simulink model "closeloop2PIBC"  (R2021a)
settings: Solver=VariableStepAuto  StartTime=0.0  StopTime=0.5  FixedStep=1e-7  MaxStep=1e-6  RelTol=1e-3
PreLoadFcn:
  | L=32e-6;
  | k=-1/3;
  | M=  L*k
  | %N=4 %nbre de spires
  | rL=3.34e-3;
  | V_dc=14.4;
  | C=100e-6;
  | r_load=5;
undefined symbols (not defined in the file or in its folder): plecs
settings Model: Creator=QUDUS  LastModifiedBy=qaromose
settings DebuggingCC: UnconnectedInputMsg=none  UnconnectedOutputMsg=none  UnconnectedLineMsg=none
settings ModelReferenceCC: EnableRefExpFcnMdlSchedulingChecks=off
settings RTWCC: Description=Generic Real-Time Target  GPUComputeCapability=5.0  DLArmComputeVersion=20.02.1

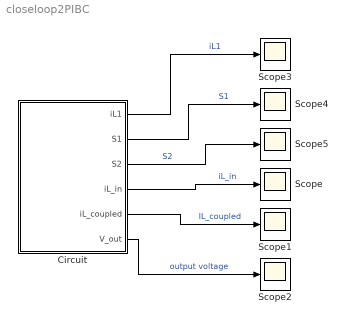
== system closeloop2PIBC ==
  Circuit : Subsystem  LoadFcn=plecs('sl', 200);  InitFcn=plecs('sl', 214);  StartFcn=plecs('sl', 208);  StopFcn=plecs('sl', 209);  mask(PlecsCircuit){PLECSData=<binary blob, 6184 chars, not shown>}
      mask prompts: PLECSData "PLECS Data (Do not delete or modify!)"
      mask init:
      | % PLACE CUSTOM INITIALIZATIONS ABOVE
      | % DO NOT REMOVE
      | plecs('sl', 215);
      | % DO NOT REMOVE
      settings: CopyFcn=plecs('sl', 203);  DeleteFcn=plecs('sl', 205);  UndoDeleteFcn=plecs('sl', 206);  PreSaveFcn=plecs('sl', 211);  PostSaveFcn=plecs('sl', 201);  NameChangeFcn=plecs('sl', 210);  DestroyFcn=plecs('sl', 207);  PreCopyFcn=plecs('sl', 216);  OpenFcn=plecs('sl', 202);  ErrorFcn=plerrorfcn
      mask Help: eval('plecs(''help'', ''qthelp:///creatingacircuit.html'')')
      mask Display: disp('PLECS\nCircuit')
  Scope{,1..5} (6 alike) : Scope
  wires:
  Circuit/5(iL_coupled) -> Scope1/1  "IL_coupled"
  Circuit/4(iL_in) -> Scope/1  "iL_in"
  Circuit/6(V_out) -> Scope2/1  "output voltage"
  Circuit/3(S2) -> Scope5/1  "S2"
  Circuit/2(S1) -> Scope4/1  "S1"
  Circuit/1(iL1) -> Scope3/1  "iL1"

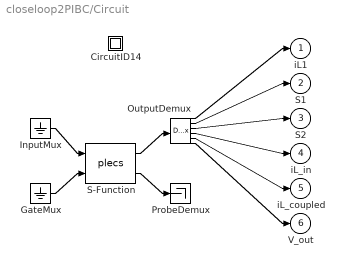
== system closeloop2PIBC/Circuit ==
  " CircuitID14 " : Subsystem
  " GateMux " : Ground
  " InputMux " : Ground
  " OutputDemux " : Demux  Outputs=[ 1 1 1 1 2 1 ]
  " ProbeDemux " : Terminator
  " S-Function " : S-Function  FunctionName=plecs  SFunctionDeploymentMode=off  EnableBusSupport=off
  iL1 : Outport  PortDimensions=1
  S1 : Outport  Port=2  PortDimensions=1
  S2 : Outport  Port=3  PortDimensions=1
  iL_in : Outport  Port=4  PortDimensions=1
  iL_coupled : Outport  Port=5  PortDimensions=2
  V_out : Outport  Port=6  PortDimensions=1
  wires:
  " InputMux "/1 -> " S-Function "/1
  " GateMux "/1 -> " S-Function "/2
  " S-Function "/1 -> " OutputDemux "/1
  " S-Function "/2 -> " ProbeDemux "/1
  " OutputDemux "/1 -> iL1/1
  " OutputDemux "/2 -> S1/1
  " OutputDemux "/3 -> S2/1
  " OutputDemux "/4 -> iL_in/1
  " OutputDemux "/5 -> iL_coupled/1
  " OutputDemux "/6 -> V_out/1

== system closeloop2PIBC/Circuit/ CircuitID14  ==
